simulink model "gm_pwm"  (R2016a)
settings: Solver=FixedStepAuto  StartTime=0.0  StopTime=.00001  FixedStep=1/100e6  RelTol=1e-3
settings Model: Creator=dskaputa  LastModifiedBy=dskaputa
settings OptimizationCC: BlockReduction=off  ConditionallyExecuteInputs=off
settings DebuggingCC: InheritedTsInSrcMsg=none
settings GRTTargetCC: GeneratePreprocessorConditionals=Use local settings

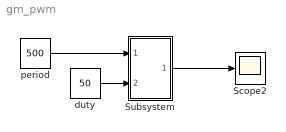
== system gm_pwm ==
  Scope2 : Scope
  Subsystem : Subsystem
  "duty " : Constant  Value=50  OutDataTypeStr=fixdt(0,27,0)  SampleTime=-1
  period : Constant  Value=500  OutDataTypeStr=fixdt(0,27,0)  SampleTime=-1
  wires:
  Subsystem/1(Out1) -> Scope2/1
  "duty "/1 -> Subsystem/2(In2)
  period/1 -> Subsystem/1(In1)

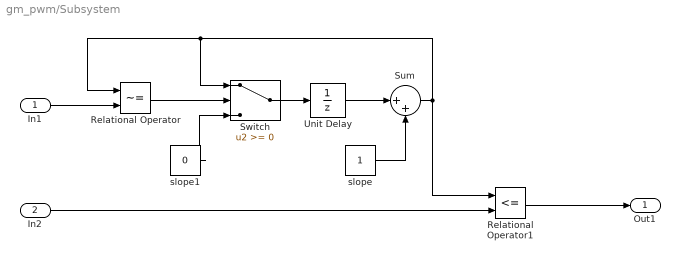
== system gm_pwm/Subsystem ==
  In1 : Inport
  In2 : Inport  Port=2
  Relational Operator : RelationalOperator  Operator=~=  OutDataTypeStr=boolean
  Relational Operator1 : RelationalOperator  Operator=<=  OutDataTypeStr=boolean
  Sum : Sum  Inputs=|++  AccumDataTypeStr=fixdt(0,27,0)  OutDataTypeStr=fixdt(0,27,0)  SaturateOnIntegerOverflow=on
  Switch : Switch
  Unit Delay : UnitDelay  SampleTime=-1
  slope : Constant  OutDataTypeStr=fixdt(0,10,0)  SampleTime=-1
  slope1 : Constant  Value=0  OutDataTypeStr=fixdt(0,10,0)  SampleTime=-1
  Out1 : Outport
  wires:
  Relational Operator/1 -> Switch/2
  In1/1 -> Relational Operator/2
  In2/1 -> Relational Operator1/2
  slope1/1 -> Switch/3
  Relational Operator1/1 -> Out1/1
  slope/1 -> Sum/2
  Unit Delay/1 -> Sum/1
  Sum/1 -> Switch/1, Relational Operator/1, Relational Operator1/1
  Switch/1 -> Unit Delay/1
